simulink model "fcsystem"  (Simulink 5.0)
settings: Solver=ode23s  StartTime=0.0  StopTime=30.0  MaxStep=0.01  RelTol=1e-5
undefined symbols (not defined in the file or in its folder): alliedsignaleff, beta0, beta1, beta2, cm_kt, cm_kv, cm_maxtorque, cm_R, Cp, cp_inertia, dc, faradays, fc_activearea, fc_anode_volume, fc_cathode_volume, fc_inlet_flow_constant, fc_numberofcells, fc_outlet_flow_constant, fcx0, gamma, hydrogengasconstant, hydrogenmolarmass, im_volume, membranedrydensity, membranedryeqvweight, membranethickness, nitrogengasconstant, nitrogenmolarmass, om_At, om_Cd, om_outlet_choke_pr, om_volume, oxygengasconstant, oxygenmolarmass, phimax0, phimax1, phimax2, phimax3, phimax4, psimax0, psimax1, psimax2, psimax3, psimax4, psimax5, R, rho, Ta, universalgasconstant, vaporgasconstant, vapormolarmass
libraries: simulink x5
(part 3 of 3)

== system fcsystem/Fuel Cell Stack System/Compressor/Compressor/Calculate Humidity Change/Saturation Pressure (Pa)1 ==
  Temperature (K) : Inport
  333.15K : Switch  Threshold=333.15  SaturateOnIntegerOverflow=on  InputSameDT=on
  433.15K : Switch  Threshold=433.15  SaturateOnIntegerOverflow=on  InputSameDT=on
  533.15K : Switch  Threshold=533.15  SaturateOnIntegerOverflow=on  InputSameDT=on
  Display{1..5} (5 alike) : Display
  Water Sat. Pressure in kPa (using 4th order approx) 333.15K<t<433.15K : Fcn  Expr=1.508306069874139e-006*u^4-0.00184416225407*u^3+0.85777718452468*u^2-1.796665242102233e+002*u+1.428163901107325e+004
  Water Sat. Pressure in kPa (using 4th order approx) 433.15<t<533.15 : Fcn  Expr=1.338811201296496e-006*u^4-0.00154136533415*u^3+0.65477998701526*u^2-1.191331991860853e+002*u+7.506492157825003e+003
  Water Sat. Pressure in kPa (using 4th order approx) t<333.15K : Fcn  Expr=6.853193243616891e-007*u^4-7.432459524835483e-004*u^3+0.30413751828818*u^2-55.61363113326989*u+3.831800671740628e+003
  Water Sat. Pressure in kPa (using 4th order approx) t>533.15K : Fcn  Expr=1.648503329422670e-6*u^4-0.00209262218193*u^3+1.01793196387371*u^2-2.241752317908023e2*u+1.878246444328017e4
  kPa to Pa : Gain  Gain=1000  SaturateOnIntegerOverflow=on
  Saturation Pressure (Pa) : Outport
  wires:
  kPa to Pa/1 -> Saturation Pressure (Pa)/1
  Water Sat. Pressure in kPa (using 4th order approx) t>533.15K/1 -> 533.15K/1
  Water Sat. Pressure in kPa (using 4th order approx) 433.15<t<533.15/1 -> 433.15K/1
  Water Sat. Pressure in kPa (using 4th order approx) 333.15K<t<433.15K/1 -> 333.15K/1
  333.15K/1 -> 433.15K/3, Display1/1
  433.15K/1 -> 533.15K/3, Display2/1
  Water Sat. Pressure in kPa (using 4th order approx) t<333.15K/1 -> 333.15K/3, Display3/1
  533.15K/1 -> kPa to Pa/1, Display4/1
  Temperature (K)/1 -> Water Sat. Pressure in kPa (using 4th order approx) t>533.15K/1, Water Sat. Pressure in kPa (using 4th order approx) 433.15<t<533.15/1, Water Sat. Pressure in kPa (using 4th order approx) 333.15K<t<433.15K/1, Water Sat. Pressure in kPa (using 4th order approx) t<333.15K/1, 533.15K/2, 433.15K/2, 333.15K/2, Display5/1

== system fcsystem/Fuel Cell Stack System/Compressor/Compressor/Compressor  Map/Compressor Efficiency ==
  Flow lb/min : Inport
  Pressure Ratio : Inport  Port=2
  Look-Up Table (2-D) : Lookup2D  RowIndex=alliedsignalflow  ColumnIndex=alliedsignalpr  OutputValues=alliedsignaleff  SaturateOnIntegerOverflow=on  InputSameDT=on
  Efficiency : Outport
  wires:
  Look-Up Table (2-D)/1 -> Efficiency/1
  Pressure Ratio/1 -> Look-Up Table (2-D)/2
  Flow lb/min/1 -> Look-Up Table (2-D)/1

== system fcsystem/Fuel Cell Stack System/Compressor/Compressor/Compressor  Map/Jensen&Kristensen Compressor Map ==
  note: SAE 1999-01-0908
  Pressure Ratio : Inport
  Corrected Speed (rpm) : Inport  Port=2
  1 Phi 2 Uc : Mux  Inputs=2
  "1 Psi 2 phimax 3 beta 4 psimax " : Mux
  Flowkg : Fcn  Expr=u[1]*rho*pi/4*dc*dc*u[2]
  Ma : Fcn  Expr=u/sqrt(gamma*R*Ta)
  Mux : Mux  Inputs=2
  Phi : Fcn  Expr=u[2]*(1-exp(u[3]*(u[1]/u[4]-1)))
  Psi : Fcn  Expr=Cp*Ta*(u[1]^((gamma-1)/gamma)-1)/0.5/u[2]/u[2]
  Uc : Fcn  Expr=pi*dc*u/60
  beta : Fcn  Expr=beta2*u^2+beta1*u+beta0
  phimax : Fcn  Expr=phimax4*u^4+phimax3*u^3+phimax2*u^2+phimax1*u+phimax0
  psimax : Fcn  Expr=psimax5*u^5+psimax4*u^4+psimax3*u^3+psimax2*u^2+psimax1*u+psimax0
  Air Flow (kg/sec) : Outport
  wires:
  Psi/1 -> "1 Psi 2 phimax 3 beta 4 psimax "/1
  psimax/1 -> "1 Psi 2 phimax 3 beta 4 psimax "/4
  "1 Psi 2 phimax 3 beta 4 psimax "/1 -> Phi/1
  Phi/1 -> 1 Phi 2 Uc/1
  beta/1 -> "1 Psi 2 phimax 3 beta 4 psimax "/3
  phimax/1 -> "1 Psi 2 phimax 3 beta 4 psimax "/2
  Flowkg/1 -> Air Flow (kg/sec)/1
  1 Phi 2 Uc/1 -> Flowkg/1
  Ma/1 -> phimax/1, beta/1, psimax/1
  Mux/1 -> Psi/1
  Uc/1 -> 1 Phi 2 Uc/2, Mux/2, Ma/1
  Pressure Ratio/1 -> Mux/1
  Corrected Speed (rpm)/1 -> Uc/1

== system fcsystem/Fuel Cell Stack System/Stack/Anode Mass Flow Model/Water Balance/Saturation Pressure (Pa) ==
  Temperature (K) : Inport
  333.15K : Switch  Threshold=333.15  SaturateOnIntegerOverflow=on  InputSameDT=on
  433.15K : Switch  Threshold=433.15  SaturateOnIntegerOverflow=on  InputSameDT=on
  533.15K : Switch  Threshold=533.15  SaturateOnIntegerOverflow=on  InputSameDT=on
  Water Sat. Pressure in kPa (using 4th order approx) 333.15K<t<433.15K : Fcn  Expr=1.508306069874139e-006*u^4-0.00184416225407*u^3+0.85777718452468*u^2-1.796665242102233e+002*u+1.428163901107325e+004
  Water Sat. Pressure in kPa (using 4th order approx) 433.15<t<533.15 : Fcn  Expr=1.338811201296496e-006*u^4-0.00154136533415*u^3+0.65477998701526*u^2-1.191331991860853e+002*u+7.506492157825003e+003
  Water Sat. Pressure in kPa (using 4th order approx) t<333.15K : Fcn  Expr=6.853193243616891e-007*u^4-7.432459524835483e-004*u^3+0.30413751828818*u^2-55.61363113326989*u+3.831800671740628e+003
  Water Sat. Pressure in kPa (using 4th order approx) t>533.15K : Fcn  Expr=1.648503329422670e-6*u^4-0.00209262218193*u^3+1.01793196387371*u^2-2.241752317908023e2*u+1.878246444328017e4
  kPa to Pa : Gain  Gain=1000  SaturateOnIntegerOverflow=on
  Saturation Pressure (Pa) : Outport
  wires:
  Temperature (K)/1 -> Water Sat. Pressure in kPa (using 4th order approx) t>533.15K/1, Water Sat. Pressure in kPa (using 4th order approx) 433.15<t<533.15/1, Water Sat. Pressure in kPa (using 4th order approx) 333.15K<t<433.15K/1, Water Sat. Pressure in kPa (using 4th order approx) t<333.15K/1, 533.15K/2, 433.15K/2, 333.15K/2
  533.15K/1 -> kPa to Pa/1
  kPa to Pa/1 -> Saturation Pressure (Pa)/1
  433.15K/1 -> 533.15K/3
  Water Sat. Pressure in kPa (using 4th order approx) t>533.15K/1 -> 533.15K/1
  Water Sat. Pressure in kPa (using 4th order approx) 433.15<t<533.15/1 -> 433.15K/1
  333.15K/1 -> 433.15K/3
  Water Sat. Pressure in kPa (using 4th order approx) 333.15K<t<433.15K/1 -> 333.15K/1
  Water Sat. Pressure in kPa (using 4th order approx) t<333.15K/1 -> 333.15K/3

== system fcsystem/Fuel Cell Stack System/Stack/Anode Mass Flow Model/Water Balance/Saturation Pressure (Pa)1 ==
  Temperature (K) : Inport
  333.15K : Switch  Threshold=333.15  SaturateOnIntegerOverflow=on  InputSameDT=on
  433.15K : Switch  Threshold=433.15  SaturateOnIntegerOverflow=on  InputSameDT=on
  533.15K : Switch  Threshold=533.15  SaturateOnIntegerOverflow=on  InputSameDT=on
  Water Sat. Pressure in kPa (using 4th order approx) 333.15K<t<433.15K : Fcn  Expr=1.508306069874139e-006*u^4-0.00184416225407*u^3+0.85777718452468*u^2-1.796665242102233e+002*u+1.428163901107325e+004
  Water Sat. Pressure in kPa (using 4th order approx) 433.15<t<533.15 : Fcn  Expr=1.338811201296496e-006*u^4-0.00154136533415*u^3+0.65477998701526*u^2-1.191331991860853e+002*u+7.506492157825003e+003
  Water Sat. Pressure in kPa (using 4th order approx) t<333.15K : Fcn  Expr=6.853193243616891e-007*u^4-7.432459524835483e-004*u^3+0.30413751828818*u^2-55.61363113326989*u+3.831800671740628e+003
  Water Sat. Pressure in kPa (using 4th order approx) t>533.15K : Fcn  Expr=1.648503329422670e-6*u^4-0.00209262218193*u^3+1.01793196387371*u^2-2.241752317908023e2*u+1.878246444328017e4
  kPa to Pa : Gain  Gain=1000  SaturateOnIntegerOverflow=on
  Saturation Pressure (Pa) : Outport
  wires:
  Water Sat. Pressure in kPa (using 4th order approx) t<333.15K/1 -> 333.15K/3
  Water Sat. Pressure in kPa (using 4th order approx) 333.15K<t<433.15K/1 -> 333.15K/1
  333.15K/1 -> 433.15K/3
  Water Sat. Pressure in kPa (using 4th order approx) 433.15<t<533.15/1 -> 433.15K/1
  Water Sat. Pressure in kPa (using 4th order approx) t>533.15K/1 -> 533.15K/1
  433.15K/1 -> 533.15K/3
  kPa to Pa/1 -> Saturation Pressure (Pa)/1
  533.15K/1 -> kPa to Pa/1
  Temperature (K)/1 -> 333.15K/2, 433.15K/2, 533.15K/2, Water Sat. Pressure in kPa (using 4th order approx) t<333.15K/1, Water Sat. Pressure in kPa (using 4th order approx) 333.15K<t<433.15K/1, Water Sat. Pressure in kPa (using 4th order approx) 433.15<t<533.15/1, Water Sat. Pressure in kPa (using 4th order approx) t>533.15K/1

== system fcsystem/Fuel Cell Stack System/Stack/Anode Mass Flow Model/inlet flow properties to mass flow/Saturation Pressure (Pa) ==
  Temperature (K) : Inport
  333.15K : Switch  Threshold=333.15  SaturateOnIntegerOverflow=on  InputSameDT=on
  433.15K : Switch  Threshold=433.15  SaturateOnIntegerOverflow=on  InputSameDT=on
  533.15K : Switch  Threshold=533.15  SaturateOnIntegerOverflow=on  InputSameDT=on
  Water Sat. Pressure in kPa (using 4th order approx) 333.15K<t<433.15K : Fcn  Expr=1.508306069874139e-006*u^4-0.00184416225407*u^3+0.85777718452468*u^2-1.796665242102233e+002*u+1.428163901107325e+004
  Water Sat. Pressure in kPa (using 4th order approx) 433.15<t<533.15 : Fcn  Expr=1.338811201296496e-006*u^4-0.00154136533415*u^3+0.65477998701526*u^2-1.191331991860853e+002*u+7.506492157825003e+003
  Water Sat. Pressure in kPa (using 4th order approx) t<333.15K : Fcn  Expr=6.853193243616891e-007*u^4-7.432459524835483e-004*u^3+0.30413751828818*u^2-55.61363113326989*u+3.831800671740628e+003
  Water Sat. Pressure in kPa (using 4th order approx) t>533.15K : Fcn  Expr=1.648503329422670e-6*u^4-0.00209262218193*u^3+1.01793196387371*u^2-2.241752317908023e2*u+1.878246444328017e4
  kPa to Pa : Gain  Gain=1000  SaturateOnIntegerOverflow=on
  Saturation Pressure (Pa) : Outport
  wires:
  Temperature (K)/1 -> Water Sat. Pressure in kPa (using 4th order approx) t>533.15K/1, Water Sat. Pressure in kPa (using 4th order approx) 433.15<t<533.15/1, Water Sat. Pressure in kPa (using 4th order approx) 333.15K<t<433.15K/1, Water Sat. Pressure in kPa (using 4th order approx) t<333.15K/1, 533.15K/2, 433.15K/2, 333.15K/2
  533.15K/1 -> kPa to Pa/1
  kPa to Pa/1 -> Saturation Pressure (Pa)/1
  433.15K/1 -> 533.15K/3
  Water Sat. Pressure in kPa (using 4th order approx) t>533.15K/1 -> 533.15K/1
  Water Sat. Pressure in kPa (using 4th order approx) 433.15<t<533.15/1 -> 433.15K/1
  333.15K/1 -> 433.15K/3
  Water Sat. Pressure in kPa (using 4th order approx) 333.15K<t<433.15K/1 -> 333.15K/1
  Water Sat. Pressure in kPa (using 4th order approx) t<333.15K/1 -> 333.15K/3

== system fcsystem/Fuel Cell Stack System/Stack/Anode Mass Flow Model/outlet flow properties to mass flow/Saturation Pressure (Pa) ==
  Temperature (K) : Inport
  333.15K : Switch  Threshold=333.15  SaturateOnIntegerOverflow=on  InputSameDT=on
  433.15K : Switch  Threshold=433.15  SaturateOnIntegerOverflow=on  InputSameDT=on
  533.15K : Switch  Threshold=533.15  SaturateOnIntegerOverflow=on  InputSameDT=on
  Water Sat. Pressure in kPa (using 4th order approx) 333.15K<t<433.15K : Fcn  Expr=1.508306069874139e-006*u^4-0.00184416225407*u^3+0.85777718452468*u^2-1.796665242102233e+002*u+1.428163901107325e+004
  Water Sat. Pressure in kPa (using 4th order approx) 433.15<t<533.15 : Fcn  Expr=1.338811201296496e-006*u^4-0.00154136533415*u^3+0.65477998701526*u^2-1.191331991860853e+002*u+7.506492157825003e+003
  Water Sat. Pressure in kPa (using 4th order approx) t<333.15K : Fcn  Expr=6.853193243616891e-007*u^4-7.432459524835483e-004*u^3+0.30413751828818*u^2-55.61363113326989*u+3.831800671740628e+003
  Water Sat. Pressure in kPa (using 4th order approx) t>533.15K : Fcn  Expr=1.648503329422670e-6*u^4-0.00209262218193*u^3+1.01793196387371*u^2-2.241752317908023e2*u+1.878246444328017e4
  kPa to Pa : Gain  Gain=1000  SaturateOnIntegerOverflow=on
  Saturation Pressure (Pa) : Outport
  wires:
  Temperature (K)/1 -> Water Sat. Pressure in kPa (using 4th order approx) t>533.15K/1, Water Sat. Pressure in kPa (using 4th order approx) 433.15<t<533.15/1, Water Sat. Pressure in kPa (using 4th order approx) 333.15K<t<433.15K/1, Water Sat. Pressure in kPa (using 4th order approx) t<333.15K/1, 533.15K/2, 433.15K/2, 333.15K/2
  533.15K/1 -> kPa to Pa/1
  kPa to Pa/1 -> Saturation Pressure (Pa)/1
  433.15K/1 -> 533.15K/3
  Water Sat. Pressure in kPa (using 4th order approx) t>533.15K/1 -> 533.15K/1
  Water Sat. Pressure in kPa (using 4th order approx) 433.15<t<533.15/1 -> 433.15K/1
  333.15K/1 -> 433.15K/3
  Water Sat. Pressure in kPa (using 4th order approx) 333.15K<t<433.15K/1 -> 333.15K/1
  Water Sat. Pressure in kPa (using 4th order approx) t<333.15K/1 -> 333.15K/3

== system fcsystem/Fuel Cell Stack System/Stack/Cathode Mass Flow Model/Inlet Flow Properties to O2, N2 and Vapor Mass Flow/Saturation Pressure (Pa) ==
  Temperature (K) : Inport
  333.15K : Switch  Threshold=333.15  SaturateOnIntegerOverflow=on  InputSameDT=on
  433.15K : Switch  Threshold=433.15  SaturateOnIntegerOverflow=on  InputSameDT=on
  533.15K : Switch  Threshold=533.15  SaturateOnIntegerOverflow=on  InputSameDT=on
  Water Sat. Pressure in kPa (using 4th order approx) 333.15K<t<433.15K : Fcn  Expr=1.508306069874139e-006*u^4-0.00184416225407*u^3+0.85777718452468*u^2-1.796665242102233e+002*u+1.428163901107325e+004
  Water Sat. Pressure in kPa (using 4th order approx) 433.15<t<533.15 : Fcn  Expr=1.338811201296496e-006*u^4-0.00154136533415*u^3+0.65477998701526*u^2-1.191331991860853e+002*u+7.506492157825003e+003
  Water Sat. Pressure in kPa (using 4th order approx) t<333.15K : Fcn  Expr=6.853193243616891e-007*u^4-7.432459524835483e-004*u^3+0.30413751828818*u^2-55.61363113326989*u+3.831800671740628e+003
  Water Sat. Pressure in kPa (using 4th order approx) t>533.15K : Fcn  Expr=1.648503329422670e-6*u^4-0.00209262218193*u^3+1.01793196387371*u^2-2.241752317908023e2*u+1.878246444328017e4
  kPa to Pa : Gain  Gain=1000  SaturateOnIntegerOverflow=on
  Saturation Pressure (Pa) : Outport
  wires:
  Temperature (K)/1 -> Water Sat. Pressure in kPa (using 4th order approx) t>533.15K/1, Water Sat. Pressure in kPa (using 4th order approx) 433.15<t<533.15/1, Water Sat. Pressure in kPa (using 4th order approx) 333.15K<t<433.15K/1, Water Sat. Pressure in kPa (using 4th order approx) t<333.15K/1, 533.15K/2, 433.15K/2, 333.15K/2
  533.15K/1 -> kPa to Pa/1
  kPa to Pa/1 -> Saturation Pressure (Pa)/1
  433.15K/1 -> 533.15K/3
  Water Sat. Pressure in kPa (using 4th order approx) t>533.15K/1 -> 533.15K/1
  Water Sat. Pressure in kPa (using 4th order approx) 433.15<t<533.15/1 -> 433.15K/1
  333.15K/1 -> 433.15K/3
  Water Sat. Pressure in kPa (using 4th order approx) 333.15K<t<433.15K/1 -> 333.15K/1
  Water Sat. Pressure in kPa (using 4th order approx) t<333.15K/1 -> 333.15K/3

== system fcsystem/Fuel Cell Stack System/Stack/Cathode Mass Flow Model/Outlet Flow Properties to O2, N2 and Vapor Mass Flow/Saturation Pressure (Pa) ==
  Temperature (K) : Inport
  333.15K : Switch  Threshold=333.15  SaturateOnIntegerOverflow=on  InputSameDT=on
  433.15K : Switch  Threshold=433.15  SaturateOnIntegerOverflow=on  InputSameDT=on
  533.15K : Switch  Threshold=533.15  SaturateOnIntegerOverflow=on  InputSameDT=on
  Water Sat. Pressure in kPa (using 4th order approx) 333.15K<t<433.15K : Fcn  Expr=1.508306069874139e-006*u^4-0.00184416225407*u^3+0.85777718452468*u^2-1.796665242102233e+002*u+1.428163901107325e+004
  Water Sat. Pressure in kPa (using 4th order approx) 433.15<t<533.15 : Fcn  Expr=1.338811201296496e-006*u^4-0.00154136533415*u^3+0.65477998701526*u^2-1.191331991860853e+002*u+7.506492157825003e+003
  Water Sat. Pressure in kPa (using 4th order approx) t<333.15K : Fcn  Expr=6.853193243616891e-007*u^4-7.432459524835483e-004*u^3+0.30413751828818*u^2-55.61363113326989*u+3.831800671740628e+003
  Water Sat. Pressure in kPa (using 4th order approx) t>533.15K : Fcn  Expr=1.648503329422670e-6*u^4-0.00209262218193*u^3+1.01793196387371*u^2-2.241752317908023e2*u+1.878246444328017e4
  kPa to Pa : Gain  Gain=1000  SaturateOnIntegerOverflow=on
  Saturation Pressure (Pa) : Outport
  wires:
  Temperature (K)/1 -> Water Sat. Pressure in kPa (using 4th order approx) t>533.15K/1, Water Sat. Pressure in kPa (using 4th order approx) 433.15<t<533.15/1, Water Sat. Pressure in kPa (using 4th order approx) 333.15K<t<433.15K/1, Water Sat. Pressure in kPa (using 4th order approx) t<333.15K/1, 533.15K/2, 433.15K/2, 333.15K/2
  533.15K/1 -> kPa to Pa/1
  kPa to Pa/1 -> Saturation Pressure (Pa)/1
  433.15K/1 -> 533.15K/3
  Water Sat. Pressure in kPa (using 4th order approx) t>533.15K/1 -> 533.15K/1
  Water Sat. Pressure in kPa (using 4th order approx) 433.15<t<533.15/1 -> 433.15K/1
  333.15K/1 -> 433.15K/3
  Water Sat. Pressure in kPa (using 4th order approx) 333.15K<t<433.15K/1 -> 333.15K/1
  Water Sat. Pressure in kPa (using 4th order approx) t<333.15K/1 -> 333.15K/3

== system fcsystem/Fuel Cell Stack System/Stack/Cathode Mass Flow Model/Water Balance/Saturation Pressure (Pa) ==
  Temperature (K) : Inport
  333.15K : Switch  Threshold=333.15  SaturateOnIntegerOverflow=on  InputSameDT=on
  433.15K : Switch  Threshold=433.15  SaturateOnIntegerOverflow=on  InputSameDT=on
  533.15K : Switch  Threshold=533.15  SaturateOnIntegerOverflow=on  InputSameDT=on
  Water Sat. Pressure in kPa (using 4th order approx) 333.15K<t<433.15K : Fcn  Expr=1.508306069874139e-006*u^4-0.00184416225407*u^3+0.85777718452468*u^2-1.796665242102233e+002*u+1.428163901107325e+004
  Water Sat. Pressure in kPa (using 4th order approx) 433.15<t<533.15 : Fcn  Expr=1.338811201296496e-006*u^4-0.00154136533415*u^3+0.65477998701526*u^2-1.191331991860853e+002*u+7.506492157825003e+003
  Water Sat. Pressure in kPa (using 4th order approx) t<333.15K : Fcn  Expr=6.853193243616891e-007*u^4-7.432459524835483e-004*u^3+0.30413751828818*u^2-55.61363113326989*u+3.831800671740628e+003
  Water Sat. Pressure in kPa (using 4th order approx) t>533.15K : Fcn  Expr=1.648503329422670e-6*u^4-0.00209262218193*u^3+1.01793196387371*u^2-2.241752317908023e2*u+1.878246444328017e4
  kPa to Pa : Gain  Gain=1000  SaturateOnIntegerOverflow=on
  Saturation Pressure (Pa) : Outport
  wires:
  Temperature (K)/1 -> Water Sat. Pressure in kPa (using 4th order approx) t>533.15K/1, Water Sat. Pressure in kPa (using 4th order approx) 433.15<t<533.15/1, Water Sat. Pressure in kPa (using 4th order approx) 333.15K<t<433.15K/1, Water Sat. Pressure in kPa (using 4th order approx) t<333.15K/1, 533.15K/2, 433.15K/2, 333.15K/2
  533.15K/1 -> kPa to Pa/1
  kPa to Pa/1 -> Saturation Pressure (Pa)/1
  433.15K/1 -> 533.15K/3
  Water Sat. Pressure in kPa (using 4th order approx) t>533.15K/1 -> 533.15K/1
  Water Sat. Pressure in kPa (using 4th order approx) 433.15<t<533.15/1 -> 433.15K/1
  333.15K/1 -> 433.15K/3
  Water Sat. Pressure in kPa (using 4th order approx) 333.15K<t<433.15K/1 -> 333.15K/1
  Water Sat. Pressure in kPa (using 4th order approx) t<333.15K/1 -> 333.15K/3

== system fcsystem/Fuel Cell Stack System/Stack/Cathode Mass Flow Model/Water Balance/Saturation Pressure (Pa)1 ==
  Temperature (K) : Inport
  333.15K : Switch  Threshold=333.15  SaturateOnIntegerOverflow=on  InputSameDT=on
  433.15K : Switch  Threshold=433.15  SaturateOnIntegerOverflow=on  InputSameDT=on
  533.15K : Switch  Threshold=533.15  SaturateOnIntegerOverflow=on  InputSameDT=on
  Water Sat. Pressure in kPa (using 4th order approx) 333.15K<t<433.15K : Fcn  Expr=1.508306069874139e-006*u^4-0.00184416225407*u^3+0.85777718452468*u^2-1.796665242102233e+002*u+1.428163901107325e+004
  Water Sat. Pressure in kPa (using 4th order approx) 433.15<t<533.15 : Fcn  Expr=1.338811201296496e-006*u^4-0.00154136533415*u^3+0.65477998701526*u^2-1.191331991860853e+002*u+7.506492157825003e+003
  Water Sat. Pressure in kPa (using 4th order approx) t<333.15K : Fcn  Expr=6.853193243616891e-007*u^4-7.432459524835483e-004*u^3+0.30413751828818*u^2-55.61363113326989*u+3.831800671740628e+003
  Water Sat. Pressure in kPa (using 4th order approx) t>533.15K : Fcn  Expr=1.648503329422670e-6*u^4-0.00209262218193*u^3+1.01793196387371*u^2-2.241752317908023e2*u+1.878246444328017e4
  kPa to Pa : Gain  Gain=1000  SaturateOnIntegerOverflow=on
  Saturation Pressure (Pa) : Outport
  wires:
  Temperature (K)/1 -> Water Sat. Pressure in kPa (using 4th order approx) t>533.15K/1, Water Sat. Pressure in kPa (using 4th order approx) 433.15<t<533.15/1, Water Sat. Pressure in kPa (using 4th order approx) 333.15K<t<433.15K/1, Water Sat. Pressure in kPa (using 4th order approx) t<333.15K/1, 533.15K/2, 433.15K/2, 333.15K/2
  533.15K/1 -> kPa to Pa/1
  kPa to Pa/1 -> Saturation Pressure (Pa)/1
  433.15K/1 -> 533.15K/3
  Water Sat. Pressure in kPa (using 4th order approx) t>533.15K/1 -> 533.15K/1
  Water Sat. Pressure in kPa (using 4th order approx) 433.15<t<533.15/1 -> 433.15K/1
  333.15K/1 -> 433.15K/3
  Water Sat. Pressure in kPa (using 4th order approx) 333.15K<t<433.15K/1 -> 333.15K/1
  Water Sat. Pressure in kPa (using 4th order approx) t<333.15K/1 -> 333.15K/3
